simulink library "TestSeq_slave_lib"  (Simulink 8.1)
settings: Solver=ode45  StartTime=0.0  StopTime=10.0  RelTol=1e-3
libraries: rtio_generic_modbus x1
settings Model: Creator=ch24070  LastModifiedBy=re25624

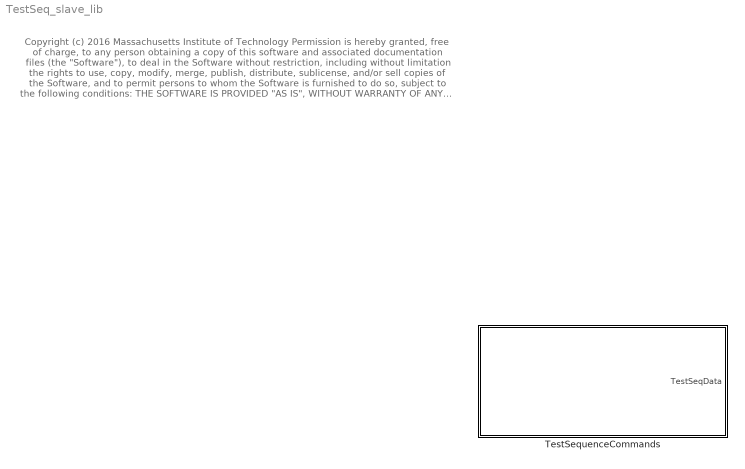
== system TestSeq_slave_lib ==
  note: Copyright (c) 2016 Massachusetts Institute of Technology
      | Permission is hereby granted, free of charge, to any person obtaining a copy of this software and associated documentation files (the "Software"), to deal
      | in the Software without restriction, including without limitation the rights to use, copy, modify, merge, publish, distribute, sublicense, and/or sell copies of the
      | Software, and to permit persons to whom the Software is furnished to do so, subject to the following conditions:
      |
      | THE SOFTWARE IS PROVIDED "AS IS", WITHOUT WARRANTY OF ANY KIND, EXPRESS OR IMPLIED, INCLUDING BUT NOT LIMITED TO THE
      | WARRANTIES OF MERCHANTABILITY, FITNESS FOR A PARTICULAR PURPOSE AND NONINFRINGEMENT. IN NO EVENT SHALL THE AUTHORS
      | OR COPYRIGHT HOLDERS BE LIABLE FOR ANY CLAIM, DAMAGES OR OTHER LIABILITY, WHETHER IN AN ACTION OF CONTRACT, TORT OR
      | OTHERWISE, ARISING FROM, OUT OF OR IN CONNECTION WITH THE SOFTWARE OR THE USE OR OTHER DEALINGS IN THE SOFTWARE
  TestSequenceCommands : Subsystem

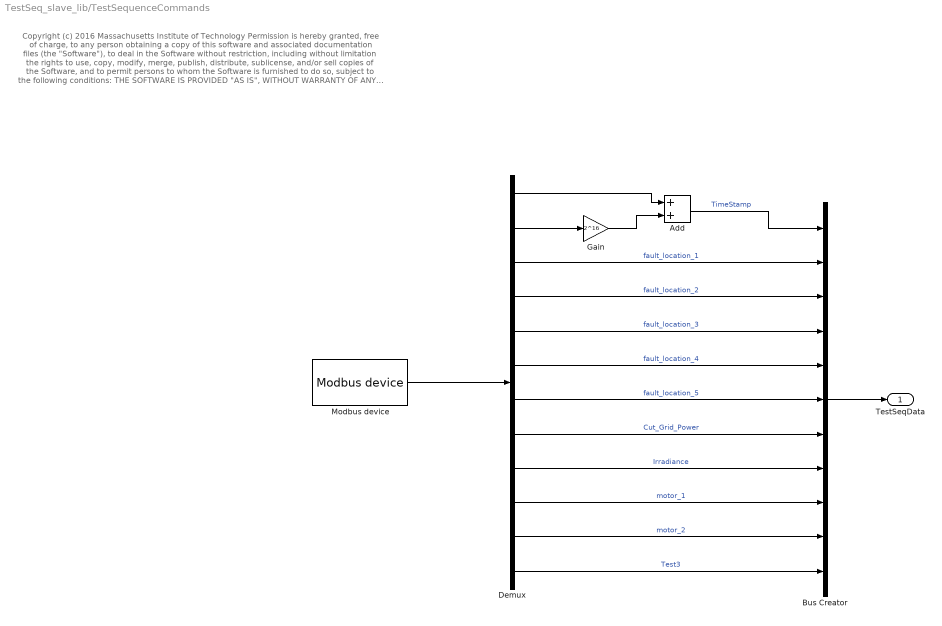
== system TestSeq_slave_lib/TestSequenceCommands ==
  note: Copyright (c) 2016 Massachusetts Institute of Technology
      | Permission is hereby granted, free of charge, to any person obtaining a copy of this software and associated documentation files (the "Software"), to deal
      | in the Software without restriction, including without limitation the rights to use, copy, modify, merge, publish, distribute, sublicense, and/or sell copies of the
      | Software, and to permit persons to whom the Software is furnished to do so, subject to the following conditions:
      |
      | THE SOFTWARE IS PROVIDED "AS IS", WITHOUT WARRANTY OF ANY KIND, EXPRESS OR IMPLIED, INCLUDING BUT NOT LIMITED TO THE
      | WARRANTIES OF MERCHANTABILITY, FITNESS FOR A PARTICULAR PURPOSE AND NONINFRINGEMENT. IN NO EVENT SHALL THE AUTHORS
      | OR COPYRIGHT HOLDERS BE LIABLE FOR ANY CLAIM, DAMAGES OR OTHER LIABILITY, WHETHER IN AN ACTION OF CONTRACT, TORT OR
      | OTHERWISE, ARISING FROM, OUT OF OR IN CONNECTION WITH THE SOFTWARE OR THE USE OR OTHER DEALINGS IN THE SOFTWARE
  Add : Sum
  Bus Creator : BusCreator  Inputs=11
  Demux : Demux  Outputs=12
  Gain : Gain  Gain=2^16
  Modbus device : rtio_generic_modbus/Modbus device  conf_name=TestSequenceCmd_cfg.opal  conf_name_mask=TestSequenceCmd_cfg.xls  sample_time=Ts
  TestSeqData : Outport
  wires:
  Bus Creator/1 -> TestSeqData/1
  Demux/11 -> Bus Creator/10  "motor_2"
  Modbus device/1 -> Demux/1
  Gain/1 -> Add/2
  Demux/2 -> Gain/1
  Demux/1 -> Add/1
  Add/1 -> Bus Creator/1  "TimeStamp"
  Demux/10 -> Bus Creator/9  "motor_1"
  Demux/9 -> Bus Creator/8  "Irradiance"
  Demux/8 -> Bus Creator/7  "Cut_Grid_Power"
  Demux/7 -> Bus Creator/6  "fault_location_5"
  Demux/6 -> Bus Creator/5  "fault_location_4"
  Demux/5 -> Bus Creator/4  "fault_location_3"
  Demux/4 -> Bus Creator/3  "fault_location_2"
  Demux/3 -> Bus Creator/2  "fault_location_1"
  Demux/12 -> Bus Creator/11  "Test3"
